simulink model "simulation6"  (R2018a)
settings: Solver=FixedStepAuto  StartTime=0.0  StopTime=1000  FixedStep=0.1  RelTol=1e-3
values from neighbouring files (symbols this model uses):
  A_w = [zeros(3,3) eye(3) ... (first row only)    [Sim4_Nolinear.m]    (also in Sim5_Nolinear.m; Sim6.m; Sim7_Nolinear.m)
  C_w = [0 1000.308 0 0 ... (first row only)    [Sim1.m]    (also in Sim3.m; Sim4_EKF.m; Sim4_Nolinear.m = [zeros(3,3) eye(3)]; Sim5_Nolinear.m = [zeros(3,3) eye(3)])
  C_wn = C_w(:,4)    [Sim1.m]    (also in Sim3.m; Sim4_EKF.m; Sim4_Nolinear.m; Sim5_Nolinear.m)
  C_wx = C_w(:,2)    [Sim1.m]    (also in Sim3.m; Sim4_EKF.m; Sim4_Nolinear.m; Sim5_Nolinear.m)
  C_wy = C_w(:,3)    [Sim1.m]    (also in Sim3.m; Sim4_EKF.m; Sim4_Nolinear.m; Sim5_Nolinear.m)
  Ce = inv(W)*Be'/(Be/W*Be')    [Sim2.m]    (also in Sim3.m; Sim4_EKF.m; Sim4_Nolinear.m; Sim5_Nolinear.m)
  D = diag([4.9e5, 4.1e6, 9.7e9])    [Sim4_EKF.m]    (also in Sim4_Nolinear.m; Sim5_Nolinear.m; Sim6.m; Sim7_Nolinear.m)
  getPos = [0;0;1]    [Sim2.m]    (also in Sim3.m; Sim4_EKF.m; Sim4_Nolinear.m; Sim5_Nolinear.m)
  getVel = [0;1;0]    [Sim2.m]    (also in Sim3.m; Sim4_EKF.m; Sim4_Nolinear.m; Sim5_Nolinear.m)
  h = 0.1    [Sim1.m]    (also in Sim2.m; Sim3.m; Sim4_EKF.m; Sim4_Nolinear.m)
  K1 = [diag([-v*k1/100000 -v*k2/1000 -v*k3]);diag([2*k4 2*k5 7.5*k6])]    [Sim4_Nolinear.m]    (also in Sim5_Nolinear.m; Sim6.m; Sim7_Nolinear.m; tf_nonlinear.m = [-1.8*diag([k1 k2 k3]);1.8*diag([k4 k5 k6])])
  K2 = diag([k4*k1 k5*k2 k6*k3])    [Sim4_Nolinear.m]    (also in Sim5_Nolinear.m; Sim6.m; Sim7_Nolinear.m; tf_nonlinear.m)
  K3 = 0.1*diag([0.01*k10,k11,k12])    [Sim4_Nolinear.m]    (also in Sim5_Nolinear.m; Sim6.m; Sim7_Nolinear.m; tf_nonlinear.m = 0.1*diag([k10,k11,k12]))
  K4 = diag([k10 k11 k12])    [Sim4_Nolinear.m]    (also in Sim5_Nolinear.m; Sim6.m; Sim7_Nolinear.m; tf_nonlinear.m)
  Kd = 7*[2*M3(1)*Omega 0 0; 0 3*M3(2,2)*Omega 0; 0 0 20*M(3,3)*Omega]    [Sim2.m]    (also in Sim3.m; Sim4_EKF.m; Sim4_Nolinear.m; Sim5_Nolinear.m = 7*[30*M3(1)*Omega 0 0; 0 150*M3(2,2)*Omega 0; 0 0 30*M(3,3)*)
  Ki = 100*(omega/10)*[M3(1)*omega^2 0 0;0 0.05*M3(2,2)*omega^2 0; 0 0 M3(3,3)*omega^2 ]*2    [Sim2.m]    (also in Sim3.m; Sim4_EKF.m; Sim4_Nolinear.m; Sim5_Nolinear.m = 10*(omega/10)*[30*M3(1)*omega^2 0 0;0 150*M3(2,2)*omega^2 0;)
  Kp = 50*[6*M3(1)*omega^2 0 0;0 M3(2,2)*omega^2 0; 0 0 10*M3(3,3)*omega^2 ]    [Sim2.m]    (also in Sim3.m; Sim4_EKF.m; Sim4_Nolinear.m; Sim5_Nolinear.m = 5*[60*M3(1)*omega^2 0 0;0 800*M3(2,2)*omega^2 0; 0 0 30*M3(3)
  M = inv(vesselABC.Minv)    [Sim1.m]    (also in Sim2.m; Sim3.m; Sim4_EKF.m = diag([2.6e7,3.6e7,7.2e10]); Sim4_Nolinear.m = diag([2.6e7,3.6e7,7.2e10]))
  mu2_c = 0.001    [Sim1.m]    (also in Sim3.m; Sim4_EKF.m; Sim4_Nolinear.m; Sim5_Nolinear.m)
  mu2_w = 0.001    [Sim1.m]    (also in Sim3.m; Sim4_EKF.m; Sim4_Nolinear.m; Sim5_Nolinear.m)
  mu_w = 0.001    [Sim1.m]    (also in Sim3.m; Sim4_EKF.m; Sim4_Nolinear.m; Sim5_Nolinear.m)
  Omega = 2*damping*omega    [Sim2.m]    (also in Sim3.m; Sim4_EKF.m; Sim4_Nolinear.m = diag([omega_1,omega_2,omega_3]); Sim5_Nolinear.m = diag([omega_1,omega_2,omega_3]))
  omega = omegab/sqrt(1-2*damping^2+sqrt(4*damping^4-4*damping^2+2))    [Sim2.m]    (also in Sim3.m; Sim4_EKF.m; Sim4_Nolinear.m; Sim5_Nolinear.m)
  phi_c = -pi/2    (= -1.57079632679)    [Sim1.m]    (also in Sim3.m; Sim4_EKF.m; Sim4_Nolinear.m; Sim5_Nolinear.m)
  psi_r = C_w(:,1)    [Sim1.m]    (also in Sim3.m; Sim4_EKF.m; Sim4_Nolinear.m; Sim5_Nolinear.m)
  rotationspeed_3 = 4*pi    (= 12.5663706144)    [Sim2.m]    (also in Sim3.m; Sim4_EKF.m; Sim4_Nolinear.m; Sim5_Nolinear.m)
  rotationspeed_5 = 4*pi    (= 12.5663706144)    [Sim2.m]    (also in Sim3.m; Sim4_EKF.m; Sim4_Nolinear.m; Sim5_Nolinear.m)
  rotationspeed_6 = 4*pi    (= 12.5663706144)    [Sim2.m]    (also in Sim3.m; Sim4_EKF.m; Sim4_Nolinear.m; Sim5_Nolinear.m)
  T = diag([100000 1000 1000])    [Sim4_Nolinear.m]    (also in Sim5_Nolinear.m; Sim6.m; Sim7_Nolinear.m; tf_nonlinear.m = 1000*diag([1 1 1]))
  thrust_1 = 420000    [Sim2.m]    (also in Sim3.m; Sim4_EKF.m; Sim4_Nolinear.m; Sim5_Nolinear.m)
  thrust_2 = 420000    [Sim2.m]    (also in Sim3.m; Sim4_EKF.m; Sim4_Nolinear.m; Sim5_Nolinear.m)
  thrust_3 = 500000    [Sim2.m]    (also in Sim3.m; Sim4_EKF.m; Sim4_Nolinear.m; Sim5_Nolinear.m)
  thrust_4 = 260000    [Sim2.m]    (also in Sim3.m; Sim4_EKF.m; Sim4_Nolinear.m; Sim5_Nolinear.m)
  thrust_5 = 1100000    [Sim2.m]    (also in Sim3.m; Sim4_EKF.m; Sim4_Nolinear.m; Sim5_Nolinear.m)
  thrust_6 = 1100000    [Sim2.m]    (also in Sim3.m; Sim4_EKF.m; Sim4_Nolinear.m; Sim5_Nolinear.m)
  thrustrate_1 = 420000/8    (= 52500)    [Sim2.m]    (also in Sim3.m; Sim4_EKF.m; Sim4_Nolinear.m; Sim5_Nolinear.m)
  thrustrate_2 = 420000/8    (= 52500)    [Sim2.m]    (also in Sim3.m; Sim4_EKF.m; Sim4_Nolinear.m; Sim5_Nolinear.m)
  thrustrate_3 = 500000/8    (= 62500)    [Sim2.m]    (also in Sim3.m; Sim4_EKF.m; Sim4_Nolinear.m; Sim5_Nolinear.m)
  thrustrate_4 = 260000/8    (= 32500)    [Sim2.m]    (also in Sim3.m; Sim4_EKF.m; Sim4_Nolinear.m; Sim5_Nolinear.m)
  thrustrate_5 = 1100000/12    (= 91666.6666667)    [Sim2.m]    (also in Sim3.m; Sim4_EKF.m; Sim4_Nolinear.m; Sim5_Nolinear.m)
  thrustrate_6 = 1100000/12    (= 91666.6666667)    [Sim2.m]    (also in Sim3.m; Sim4_EKF.m; Sim4_Nolinear.m; Sim5_Nolinear.m)
  V_mean = 0.5    [Sim1.m]    (also in Sim3.m; Sim4_EKF.m; Sim4_Nolinear.m; Sim5_Nolinear.m)
  W_gust = Ug    [Sim1.m]    (also in Sim3.m; Sim4_EKF.m; Sim4_Nolinear.m; Sim5_Nolinear.m)
  W_mean = 15    [Sim1.m]    (also in Sim3.m; Sim4_EKF.m; Sim4_Nolinear.m; Sim5_Nolinear.m)
  xposition = [77, 74, 70, -65, -72, -72]    [Sim2.m]    (also in Sim3.m; Sim4_EKF.m; Sim4_Nolinear.m; Sim5_Nolinear.m)
  yposition = [0, 0, 0, 0, 5, -5]    [Sim2.m]    (also in Sim3.m; Sim4_EKF.m; Sim4_Nolinear.m; Sim5_Nolinear.m)
undefined symbols (not defined in the file or in its folder): Hoerner, magnitude, sigbuilder_block, vessel
libraries: simulink x3, marine_hydro x2, marine_gnc x1, simulink_extras x1
settings Model: SimulationMode=accelerator  Creator=jonbjor  LastModifiedBy=Shuyuan

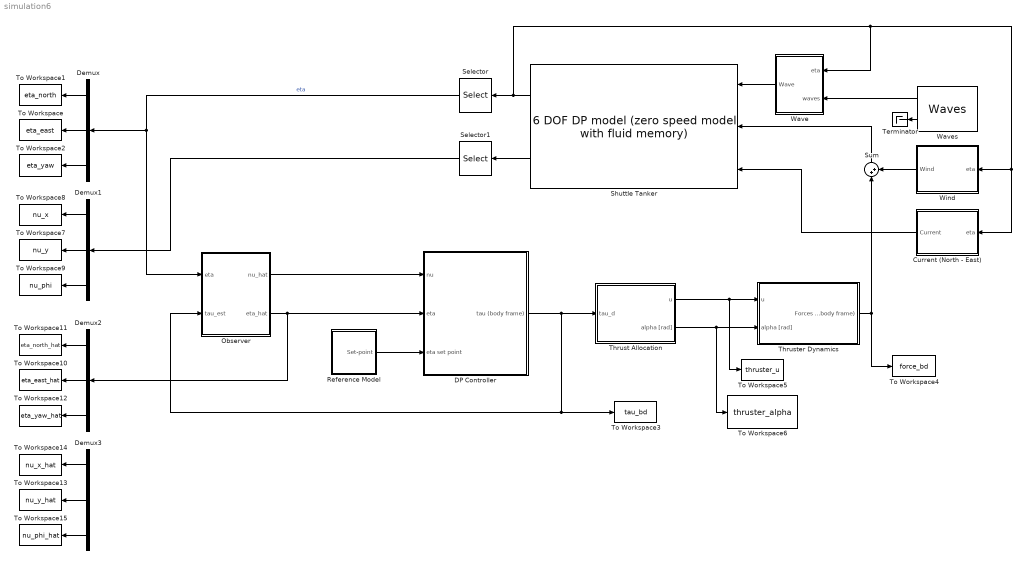
== system simulation6 ==
  Current (North - East) : Subsystem
  DP Controller : Subsystem
  Demux{,1..3} (4 alike) : Demux  Outputs=3
  Observer : Subsystem
  Reference Model : Subsystem
  Selector : Selector  InputPortWidth=6  IndexOptions=Index vector (dialog)  Indices=[1 2 6]  OutputSizes=1
  Selector1 : Selector  InputPortWidth=6  IndexOptions=Index vector (dialog)  Indices=[1 2 6]  OutputSizes=1
  Shuttle Tanker : marine_hydro/Hydro Library/6 DOF DP model  (zero speed model with fluid memory)  ABC=vesselABC  rho=1025  Axc=0.9*vessel.main.T*vessel.main.B  Ayc=0.9*vessel.main.T*vessel.main.Lpp  CX=1  CY_2D=Hoerner(vessel.main.B,vessel.main.T)  Bv=vessel.Bv  mask(6 DOF zero speed model){}
      link override "Integrator1 ": InitialCondition=nu0
      link override Integrator2: InitialCondition=eta0
      settings: SourceProductName=MSS Hydro
      mask Display:
      | image('shuttleTanker.jpg');
      | color('white'); port_label('output', 1, 'eta')
      | color('white'); port_label('output', 2, 'nu')
      | color('white'); port_label('input', 1, 'tau_wave')
      | color('white'); port_label('input', 2, 'tau')
      | color('white'); port_label('input', 3, 'nu_c')
  Sum : Sum  Inputs=|++
  Terminator : Terminator
  Thrust Allocation : Subsystem
  Thruster Dynamics : Subsystem  mask{thrusterfault=off}
      mask prompts: thrusterfault "Fault on thruster #2 and #5?"
  To Workspace : ToWorkspace  VariableName=eta_east  SaveFormat=Timeseries  SampleTime=-1
  To Workspace1 : ToWorkspace  VariableName=eta_north  SaveFormat=Timeseries  SampleTime=-1
  To Workspace10 : ToWorkspace  VariableName=eta_east_hat  SaveFormat=Timeseries  SampleTime=-1
  To Workspace11 : ToWorkspace  VariableName=eta_north_hat  SaveFormat=Timeseries  SampleTime=-1
  To Workspace12 : ToWorkspace  VariableName=eta_yaw_hat  SaveFormat=Timeseries  SampleTime=-1
  To Workspace13 : ToWorkspace  VariableName=nu_y_hat  SaveFormat=Timeseries  SampleTime=-1
  To Workspace14 : ToWorkspace  VariableName=nu_x_hat  SaveFormat=Timeseries  SampleTime=-1
  To Workspace15 : ToWorkspace  VariableName=nu_phi_hat  SaveFormat=Timeseries  SampleTime=-1
  To Workspace2 : ToWorkspace  VariableName=eta_yaw  SaveFormat=Timeseries  SampleTime=-1
  To Workspace3 : ToWorkspace  VariableName=tau_bd  SaveFormat=Timeseries  SampleTime=-1
  To Workspace4 : ToWorkspace  VariableName=force_bd  SaveFormat=Timeseries  SampleTime=-1
  To Workspace5 : ToWorkspace  VariableName=thruster_u  SaveFormat=Timeseries  SampleTime=-1
  To Workspace6 : ToWorkspace  VariableName=thruster_alpha  SaveFormat=Timeseries  SampleTime=-1
  To Workspace7 : ToWorkspace  VariableName=nu_y  SaveFormat=Timeseries  SampleTime=-1
  To Workspace8 : ToWorkspace  VariableName=nu_x  SaveFormat=Timeseries  SampleTime=-1
  To Workspace9 : ToWorkspace  VariableName=nu_phi  SaveFormat=Timeseries  SampleTime=-1
  Wave : Subsystem  mask{waveforces=on}
      mask prompts: waveforces "Waveforces enabled"
  Waves : marine_gnc/Environment/Waves/Waves  spectrum_type=ITTC  disp_flag=on  plot_spectrum=off  plot_realization=off  hs=5  omega_peak=2*pi/10  psi_mean=350*2*pi/360  gamma=-1  spread=2  depth=inf  nfreq=20  ndir=10  energylim=0.005  freq_cutoff=3  dir_cutoff=0  rand_seed=123  rand_freq=on  rand_dir=on  Zeta_a=0  Omega=0  Phase=0  Wavenum=0  Psi=0
      settings: SourceProductName=MSS GNC
  Wind : Subsystem
  wires:
  Shuttle Tanker/2 -> Selector1/1
  Reference Model/1(Set-point) -> DP Controller/3(eta set point)
  Shuttle Tanker/1 -> Selector/1, Current (North - East)/1(eta), Wind/1(eta), Wave/1(eta)
  Wave/1(Wave) -> Shuttle Tanker/1
  Waves/1 -> Wave/2(waves)
  Waves/2 -> Terminator/1
  Thrust Allocation/1(u) -> To Workspace5/1, Thruster Dynamics/1(u)
  Wind/1(Wind) -> Sum/2
  Thruster Dynamics/1("Forces (body frame) ") -> Sum/1, To Workspace4/1
  Sum/1 -> Shuttle Tanker/2
  Thrust Allocation/2(alpha [rad]) -> To Workspace6/1, Thruster Dynamics/2(alpha [rad])
  Demux/3 -> To Workspace2/1
  Selector/1 -> Observer/1(eta), Demux/1  "eta"
  Demux/1 -> To Workspace1/1
  Demux/2 -> To Workspace/1
  Current (North - East)/1(Current) -> Shuttle Tanker/3
  DP Controller/1(tau (body frame)) -> Observer/2(tau_est), To Workspace3/1, Thrust Allocation/1(tau_d)
  Demux1/1 -> To Workspace8/1
  Demux1/2 -> To Workspace7/1
  Selector1/1 -> Demux1/1
  Demux1/3 -> To Workspace9/1
  Demux3/1 -> To Workspace14/1
  Demux3/3 -> To Workspace15/1
  Demux2/1 -> To Workspace11/1
  Demux3/2 -> To Workspace13/1
  Observer/2(eta_hat) -> DP Controller/2(eta), Demux2/1
  Demux2/2 -> To Workspace10/1
  Demux2/3 -> To Workspace12/1
  Observer/1(nu_hat) -> DP Controller/1(nu)

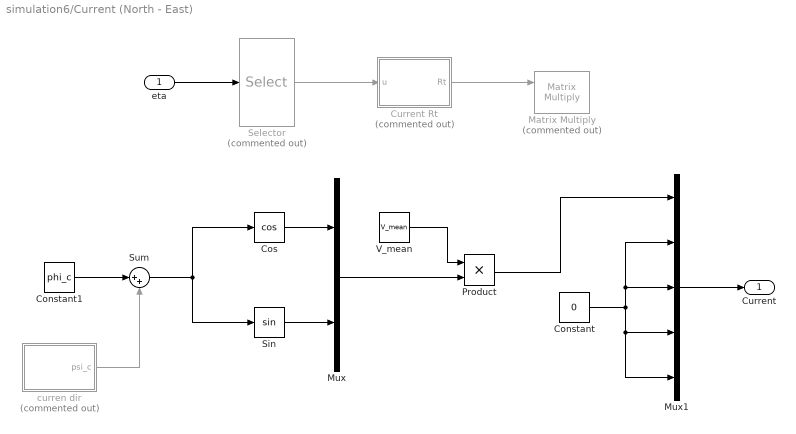
== system simulation6/Current (North - East) ==
  eta : Inport
  Constant : Constant  Value=0
  Constant1 : Constant  Value=phi_c
  Cos : Trigonometry  Operator=cos
  Current Rt : MATLAB Function  Commented=on  TreatAsAtomicUnit=on
  Matrix Multiply : Product  Commented=on  Multiplication=Matrix(*)
  Mux : Mux  Inputs=2
  Mux1 : Mux  Inputs=5
  Product : Product
  Selector : Selector  Commented=on  InputPortWidth=6  IndexOptions=Index vector (dialog)  Indices=[6]  OutputSizes=1
  Sin : Trigonometry
  Sum : Sum  Inputs=|++
  V_mean : Constant  Value=V_mean
  curren dir : Subsystem  Commented=on
  Current : Outport
  wires:
  V_mean/1 -> Product/1
  Mux1/1 -> Current/1
  Cos/1 -> Mux/1
  Mux/1 -> Product/2
  Sin/1 -> Mux/2
  Constant/1 -> Mux1/5, Mux1/4, Mux1/3, Mux1/2
  Constant1/1 -> Sum/1
  curren dir/1("psi_c ") -> Sum/2
  Sum/1 -> Sin/1, Cos/1
  eta/1 -> Selector/1
  Selector/1 -> Current Rt/1(u)
  Current Rt/1(Rt) -> Matrix Multiply/1
  Product/1 -> Mux1/1

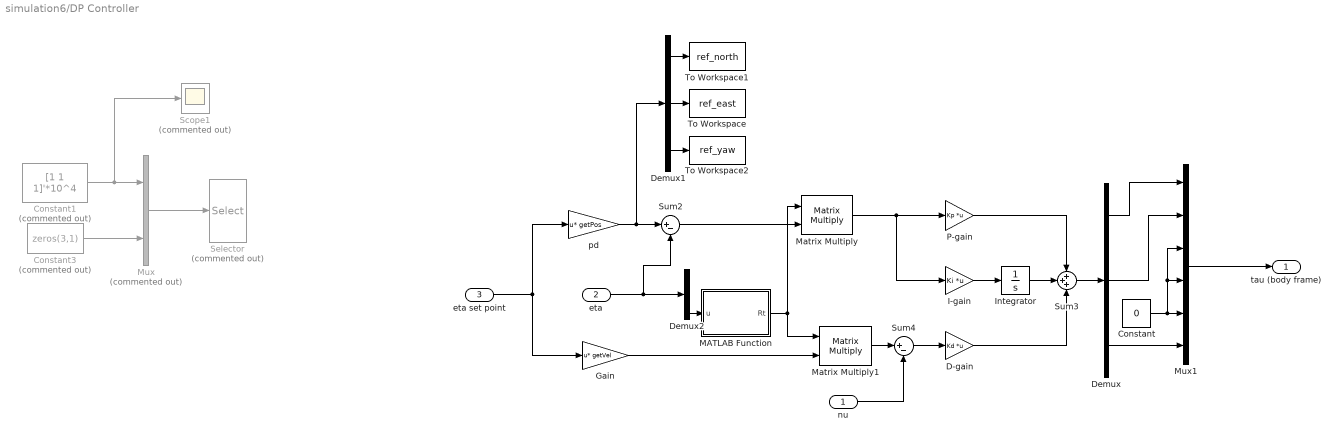
== system simulation6/DP Controller ==
  nu : Inport
  eta : Inport  Port=2
  eta set point : Inport  Port=3
  Constant : Constant  Value=0
  Constant1 : Constant  Commented=on  Value=[1 1 1]'*10^4
  Constant3 : Constant  Commented=on  Value=zeros(3,1)
  D-gain : Gain  Gain=Kd  Multiplication=Matrix(K*u)
  Demux : Demux  Outputs=3
  Demux1 : Demux  Outputs=3
  Demux2 : Demux  Outputs=3
  Gain : Gain  Gain=getVel  Multiplication=Matrix(u*K)
  I-gain : Gain  Gain=Ki  Multiplication=Matrix(K*u)
  Integrator : Integrator
  MATLAB Function : MATLAB Function  TreatAsAtomicUnit=on
  Matrix Multiply : Product  Multiplication=Matrix(*)
  Matrix Multiply1 : Product  Multiplication=Matrix(*)
  Mux : Mux  Commented=on  Inputs=2
  Mux1 : Mux  Inputs=6
  P-gain : Gain  Gain=Kp  Multiplication=Matrix(K*u)
  Scope1 : Scope  Commented=on
  Selector : Selector  Commented=on  InputPortWidth=6  IndexOptions=Index vector (dialog)  Indices=[1 2 4 5 6 3]  OutputSizes=1
  Sum2 : Sum  Inputs=|+-
  Sum3 : Sum  Inputs=+++
  Sum4 : Sum  Inputs=|+-
  To Workspace : ToWorkspace  VariableName=ref_east  SaveFormat=Timeseries  SampleTime=-1
  To Workspace1 : ToWorkspace  VariableName=ref_north  SaveFormat=Timeseries  SampleTime=-1
  To Workspace2 : ToWorkspace  VariableName=ref_yaw  SaveFormat=Timeseries  SampleTime=-1
  pd : Gain  Gain=getPos  Multiplication=Matrix(u*K)
  tau (body frame) : Outport
  wires:
  Constant1/1 -> Scope1/1, Mux/1
  Constant3/1 -> Mux/2
  Mux/1 -> Selector/1
  Sum4/1 -> D-gain/1
  I-gain/1 -> Integrator/1
  MATLAB Function/1(Rt) -> Matrix Multiply1/1, Matrix Multiply/1
  Demux/3 -> Mux1/6
  pd/1 -> Demux1/1, Sum2/1
  Demux1/1 -> To Workspace1/1
  Demux1/3 -> To Workspace2/1
  Demux/1 -> Mux1/1
  Matrix Multiply/1 -> I-gain/1, P-gain/1
  D-gain/1 -> Sum3/3
  nu/1 -> Sum4/2
  Sum2/1 -> Matrix Multiply/2
  Sum3/1 -> Demux/1
  eta/1 -> Demux2/1, Sum2/2
  Constant/1 -> Mux1/4, Mux1/3, Mux1/5
  eta set point/1 -> pd/1, Gain/1
  P-gain/1 -> Sum3/1
  Demux1/2 -> To Workspace/1
  Demux2/3 -> MATLAB Function/1(u)
  Demux/2 -> Mux1/2
  Matrix Multiply1/1 -> Sum4/1
  Gain/1 -> Matrix Multiply1/2
  Integrator/1 -> Sum3/2
  Mux1/1 -> tau (body frame)/1

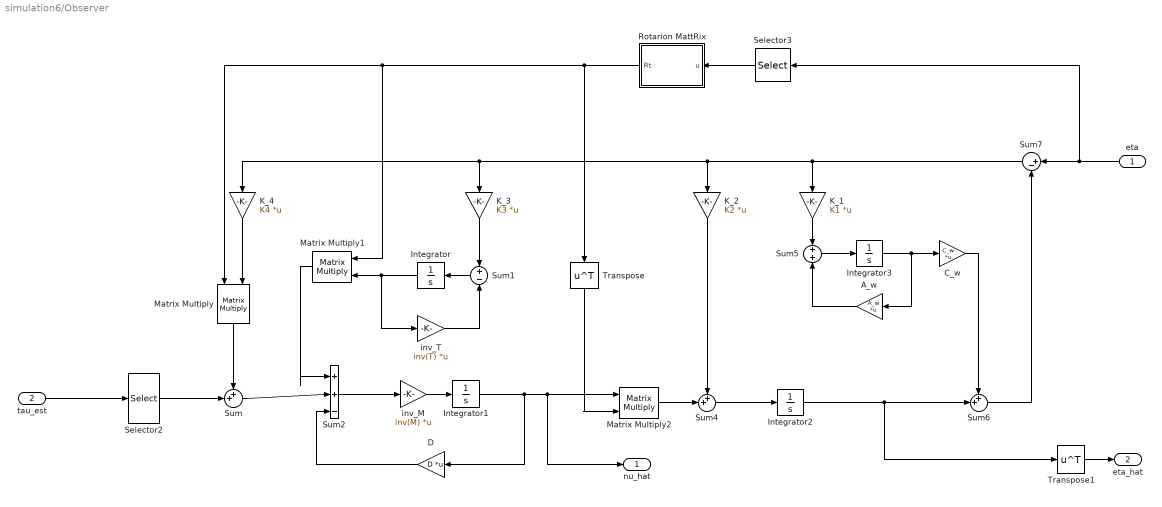
== system simulation6/Observer ==
  eta : Inport
  tau_est : Inport  Port=2
  A_w : Gain  Gain=A_w  Multiplication=Matrix(K*u)
  C_w : Gain  Gain=C_w  Multiplication=Matrix(K*u)
  D : Gain  Gain=D  Multiplication=Matrix(K*u)
  Integrator{,1..3} (4 alike) : Integrator
  K_1 : Gain  Gain=K1  Multiplication=Matrix(K*u)
  K_2 : Gain  Gain=K2  Multiplication=Matrix(K*u)
  K_3 : Gain  Gain=K3  Multiplication=Matrix(K*u)
  K_4 : Gain  Gain=K4  Multiplication=Matrix(K*u)
  Matrix Multiply : Product  Multiplication=Matrix(*)
  Matrix Multiply1 : Product  Multiplication=Matrix(*)
  Matrix Multiply2 : Product  Multiplication=Matrix(*)
  Rotarion MattRix : MATLAB Function  TreatAsAtomicUnit=on
  Selector2 : Selector  InputPortWidth=6  IndexOptions=Index vector (dialog)  Indices=[1 2 6]  OutputSizes=1
  Selector3 : Selector  InputPortWidth=3  IndexOptions=Index vector (dialog)  Indices=[3]  OutputSizes=1
  Sum : Sum  Inputs=++|
  Sum1 : Sum  Inputs=+|-
  Sum2 : Sum  Inputs=|++-
  Sum4 : Sum  Inputs=++|
  Sum5 : Sum  Inputs=+|+
  Sum6 : Sum  Inputs=++|
  Sum7 : Sum  Inputs=|+-
  Transpose : Math  Operator=transpose  SaturateOnIntegerOverflow=on
  Transpose1 : Math  Operator=transpose  SaturateOnIntegerOverflow=on
  inv_M : Gain  Gain=inv(M)  Multiplication=Matrix(K*u)
  inv_T : Gain  Gain=inv(T)  Multiplication=Matrix(K*u)
  nu_hat : Outport
  eta_hat : Outport  Port=2
  wires:
  tau_est/1 -> Selector2/1
  eta/1 -> Selector3/1, Sum7/1
  Selector3/1 -> Rotarion MattRix/1(u)
  Selector2/1 -> Sum/2
  Matrix Multiply/1 -> Sum/1
  K_4/1 -> Matrix Multiply/2
  Rotarion MattRix/1(Rt) -> Matrix Multiply/1, Matrix Multiply1/1, Transpose/1
  Sum1/1 -> Integrator/1
  K_3/1 -> Sum1/1
  Integrator/1 -> inv_T/1, Matrix Multiply1/2
  inv_T/1 -> Sum1/2
  inv_M/1 -> Integrator1/1
  Integrator1/1 -> Matrix Multiply2/1, nu_hat/1, D/1
  Sum2/1 -> inv_M/1
  D/1 -> Sum2/3
  Matrix Multiply1/1 -> Sum2/1
  Sum/1 -> Sum2/2
  K_2/1 -> Sum4/1
  Matrix Multiply2/1 -> Sum4/2
  Sum4/1 -> Integrator2/1
  Integrator3/1 -> A_w/1, C_w/1
  K_1/1 -> Sum5/1
  Sum5/1 -> Integrator3/1
  A_w/1 -> Sum5/2
  Integrator2/1 -> Transpose1/1, Sum6/2
  C_w/1 -> Sum6/1
  Sum7/1 -> K_4/1, K_3/1, K_2/1, K_1/1
  Sum6/1 -> Sum7/2
  Transpose/1 -> Matrix Multiply2/2
  Transpose1/1 -> eta_hat/1

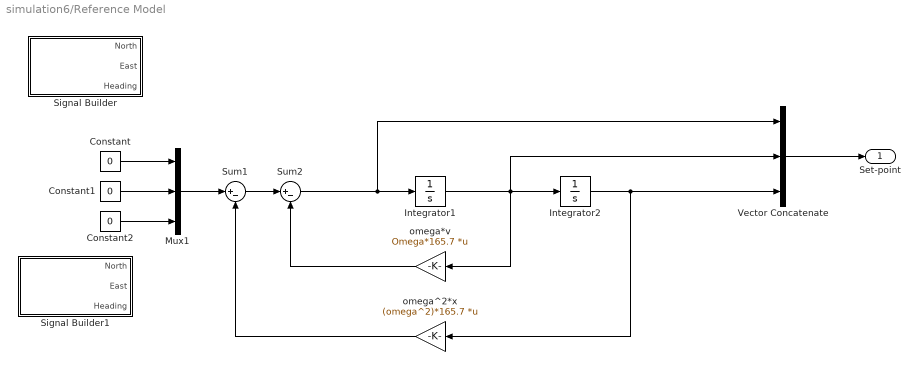
== system simulation6/Reference Model ==
  Constant : Constant  Value=0  VectorParams1D=off  SampleTime=-1
  Constant1 : Constant  Value=0  VectorParams1D=off  SampleTime=-1
  Constant2 : Constant  Value=0  VectorParams1D=off  SampleTime=-1
  Integrator1 : Integrator
  Integrator2 : Integrator
  Mux1 : Mux  Inputs=3
  Signal Builder : Subsystem  Tag=STV Subsys  LoadFcn=sigbuilder_block('load');  StartFcn=sigbuilder_block('start');  StopFcn=sigbuilder_block('stop');  ClipboardFcn=sigbuilder_block('clipboard');  mask(Sigbuilder block){tuvar=[0:10]}
      mask help: Simulink:masks:SigbuilderBlock_MD
      mask init:
      | if ~strcmp(get_param(bdroot(gcbh),'SimulationStatus'),'stopped') tuvar = sigbuilder_block('maskInit'); end
      settings: CopyFcn=sigbuilder_block('copy');  DeleteFcn=sigbuilder_block('delete');  ModelCloseFcn=sigbuilder_block('modelClose');  PreSaveFcn=sigbuilder_block('preSave');  PauseFcn=sigbuilder_block('pause');  ContinueFcn=sigbuilder_block('continue');  NameChangeFcn=sigbuilder_block('namechange');  OpenFcn=sigbuilder_block('open',[5.4 33 1141.2 516 ]);  CloseFcn=sigbuilder_block('close');
      mask Display: plot(0, 0, 100, 100,[2, 2, 32, 32, 2], [68, 8, 8, 68, 68],[32, 2], [38, 38], [32, 19, 2],[53, 60, 44], [32, 17, 17, 2],[16, 16, 31, 31]);txt = getActiveGroup(gcbh);text(2, 100, txt,'verticalAlignment', 'top');
  Signal Builder1 : Subsystem  Tag=STV Subsys  LoadFcn=sigbuilder_block('load');  StartFcn=sigbuilder_block('start');  StopFcn=sigbuilder_block('stop');  ClipboardFcn=sigbuilder_block('clipboard');  mask(Sigbuilder block){tuvar=[0:10]}
      mask help: Simulink:masks:SigbuilderBlock_MD
      mask init:
      | if ~strcmp(get_param(bdroot(gcbh),'SimulationStatus'),'stopped') tuvar = sigbuilder_block('maskInit'); end
      settings: CopyFcn=sigbuilder_block('copy');  DeleteFcn=sigbuilder_block('delete');  ModelCloseFcn=sigbuilder_block('modelClose');  PreSaveFcn=sigbuilder_block('preSave');  PauseFcn=sigbuilder_block('pause');  ContinueFcn=sigbuilder_block('continue');  NameChangeFcn=sigbuilder_block('namechange');  OpenFcn=sigbuilder_block('open',[5.4 33 1141.2 516 ]);  CloseFcn=sigbuilder_block('close');
      mask Display: plot(0, 0, 100, 100,[2, 2, 32, 32, 2], [68, 8, 8, 68, 68],[32, 2], [38, 38], [32, 19, 2],[53, 60, 44], [32, 17, 17, 2],[16, 16, 31, 31]);txt = getActiveGroup(gcbh);text(2, 100, txt,'verticalAlignment', 'top');
  Sum1 : Sum  Inputs=|+-
  Sum2 : Sum  Inputs=|+-
  Vector Concatenate : Concatenate  NumInputs=3  Mode=Multidimensional array  ConcatenateDimension=2
  omega*v : Gain  Gain=Omega*165.7  Multiplication=Matrix(K*u)
  omega^2*x : Gain  Gain=(omega^2)*165.7  Multiplication=Matrix(K*u)
  Set-point : Outport
  wires:
  omega*v/1 -> Sum2/2
  Sum1/1 -> Sum2/1
  omega^2*x/1 -> Sum1/2
  Sum2/1 -> Vector Concatenate/1, Integrator1/1
  Integrator2/1 -> omega^2*x/1, Vector Concatenate/3
  Integrator1/1 -> omega*v/1, Vector Concatenate/2, Integrator2/1
  Vector Concatenate/1 -> Set-point/1
  Mux1/1 -> Sum1/1
  Constant/1 -> Mux1/1
  Constant2/1 -> Mux1/3
  Constant1/1 -> Mux1/2

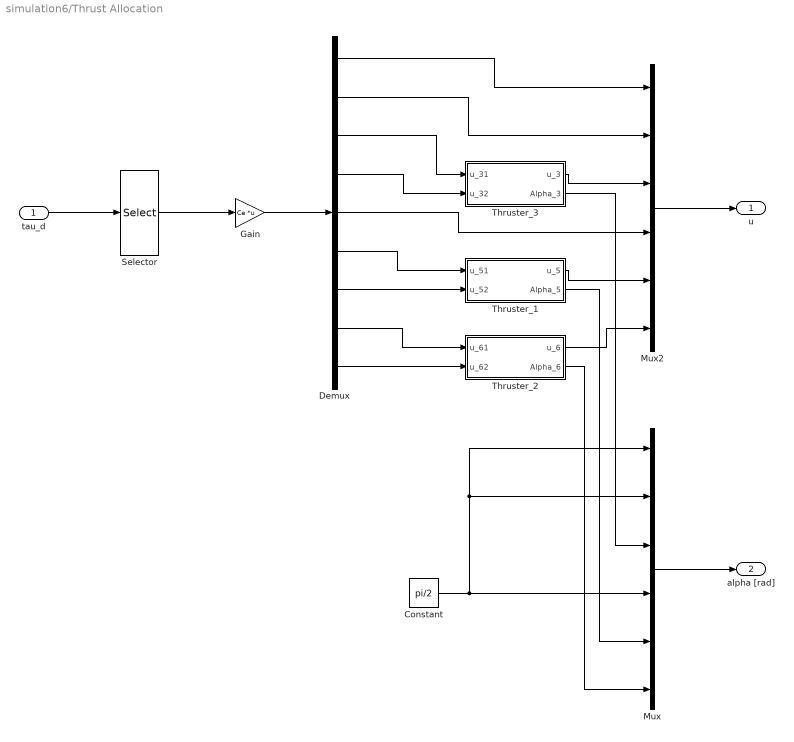
== system simulation6/Thrust Allocation ==
  tau_d : Inport
  Constant : Constant  Value=pi/2
  Demux : Demux  Outputs=9
  Gain : Gain  Gain=Ce  Multiplication=Matrix(K*u)
  Mux : Mux  Inputs=6
  Mux2 : Mux  Inputs=6
  Selector : Selector  InputPortWidth=6  IndexOptions=Index vector (dialog)  Indices=[1 2 6]  OutputSizes=1
  Thruster_1 : Subsystem
  Thruster_2 : Subsystem
  Thruster_3 : Subsystem
  u : Outport
  alpha [rad] : Outport  Port=2
  wires:
  tau_d/1 -> Selector/1
  Constant/1 -> Mux/4, Mux/2, Mux/1
  Mux/1 -> alpha [rad]/1
  Gain/1 -> Demux/1
  Mux2/1 -> u/1
  Demux/1 -> Mux2/1
  Demux/2 -> Mux2/2
  Demux/5 -> Mux2/4
  Demux/3 -> Thruster_3/1(u_31)
  Demux/4 -> Thruster_3/2(u_32)
  Thruster_3/1(u_3) -> Mux2/3
  Thruster_1/1(u_5) -> Mux2/5
  Thruster_2/1(u_6) -> Mux2/6
  Demux/6 -> Thruster_1/1(u_51)
  Demux/7 -> Thruster_1/2(u_52)
  Demux/8 -> Thruster_2/1(u_61)
  Demux/9 -> Thruster_2/2(u_62)
  Thruster_3/2(Alpha_3) -> Mux/3
  Thruster_1/2(Alpha_5) -> Mux/5
  Thruster_2/2(Alpha_6) -> Mux/6
  Selector/1 -> Gain/1

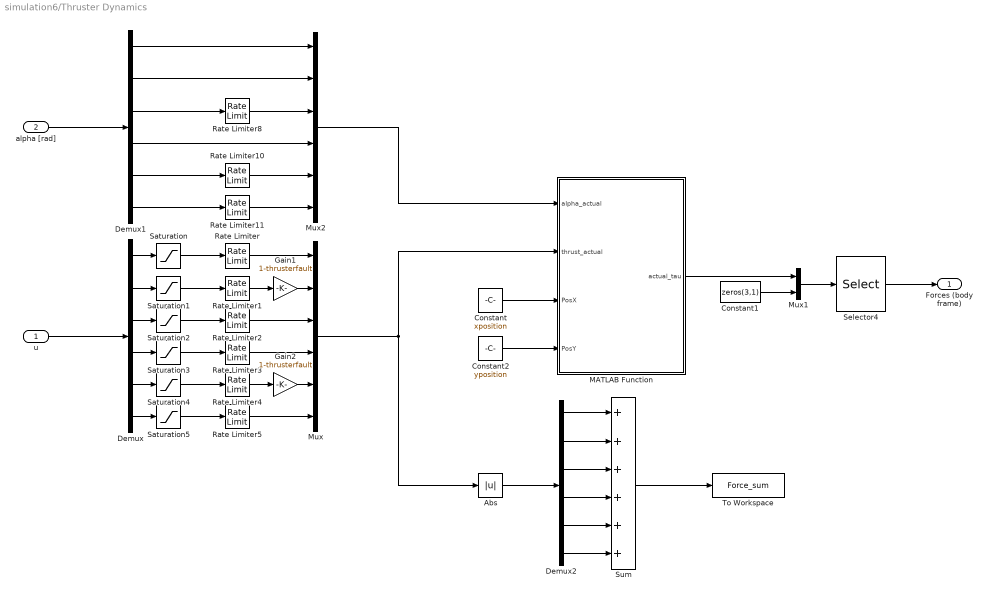
== system simulation6/Thruster Dynamics ==
  u : Inport
  alpha [rad] : Inport  Port=2
  Abs : Abs
  Constant : Constant  Value=xposition
  Constant1 : Constant  Value=zeros(3,1)
  Constant2 : Constant  Value=yposition
  Demux : Demux  Outputs=6
  Demux1 : Demux  Outputs=6
  Demux2 : Demux  Outputs=6
  Gain1 : Gain  Gain=1-thrusterfault
  Gain2 : Gain  Gain=1-thrusterfault
  MATLAB Function : MATLAB Function  TreatAsAtomicUnit=on
  Mux : Mux  Inputs=6
  Mux1 : Mux  Inputs=2
  Mux2 : Mux  Inputs=6
  Rate Limiter : RateLimiter  RisingSlewLimit=thrustrate_1  FallingSlewLimit=-thrustrate_1  SampleTimeMode=inherited
  Rate Limiter1 : RateLimiter  RisingSlewLimit=thrustrate_2  FallingSlewLimit=-thrustrate_2  SampleTimeMode=inherited
  Rate Limiter10 : RateLimiter  RisingSlewLimit=rotationspeed_5  FallingSlewLimit=-rotationspeed_5  SampleTimeMode=inherited
  Rate Limiter11 : RateLimiter  RisingSlewLimit=rotationspeed_6  FallingSlewLimit=-rotationspeed_6  SampleTimeMode=inherited
  Rate Limiter2 : RateLimiter  RisingSlewLimit=thrustrate_3  FallingSlewLimit=-thrustrate_3  SampleTimeMode=inherited
  Rate Limiter3 : RateLimiter  RisingSlewLimit=thrustrate_4  FallingSlewLimit=-thrustrate_4  SampleTimeMode=inherited
  Rate Limiter4 : RateLimiter  RisingSlewLimit=thrustrate_5  FallingSlewLimit=-thrustrate_5  SampleTimeMode=inherited
  Rate Limiter5 : RateLimiter  RisingSlewLimit=thrustrate_6  FallingSlewLimit=-thrustrate_6  SampleTimeMode=inherited
  Rate Limiter8 : RateLimiter  RisingSlewLimit=rotationspeed_3  FallingSlewLimit=-rotationspeed_3  SampleTimeMode=inherited
  Saturation : Saturate  UpperLimit=thrust_1  LowerLimit=-thrust_1
  Saturation1 : Saturate  UpperLimit=thrust_2  LowerLimit=-thrust_2
  Saturation2 : Saturate  UpperLimit=thrust_3  LowerLimit=-thrust_3
  Saturation3 : Saturate  UpperLimit=thrust_4  LowerLimit=-thrust_4
  Saturation4 : Saturate  UpperLimit=thrust_5  LowerLimit=-thrust_5
  Saturation5 : Saturate  UpperLimit=thrust_6  LowerLimit=-thrust_6
  Selector4 : Selector  InputPortWidth=6  IndexOptions=Index vector (dialog)  Indices=[1 2 4 5 6 3]  OutputSizes=1
  Sum : Sum  Inputs=6
  To Workspace : ToWorkspace  VariableName=Force_sum  SaveFormat=Timeseries  SampleTime=-1
  "Forces (body frame) " : Outport
  wires:
  Rate Limiter2/1 -> Mux/3
  Saturation/1 -> Rate Limiter/1
  Mux1/1 -> Selector4/1
  Constant1/1 -> Mux1/2
  Demux/5 -> Saturation4/1
  Demux/4 -> Saturation3/1
  Saturation4/1 -> Rate Limiter4/1
  Demux/2 -> Saturation1/1
  Saturation1/1 -> Rate Limiter1/1
  Demux/1 -> Saturation/1
  Demux/3 -> Saturation2/1
  Saturation2/1 -> Rate Limiter2/1
  Saturation3/1 -> Rate Limiter3/1
  Selector4/1 -> "Forces (body frame) "/1
  Gain1/1 -> Mux/2
  Rate Limiter3/1 -> Mux/4
  Rate Limiter1/1 -> Gain1/1
  Rate Limiter/1 -> Mux/1
  Rate Limiter4/1 -> Gain2/1
  Saturation5/1 -> Rate Limiter5/1
  Demux/6 -> Saturation5/1
  Rate Limiter5/1 -> Mux/6
  Gain2/1 -> Mux/5
  Demux1/6 -> Rate Limiter11/1
  Demux1/3 -> Rate Limiter8/1
  Rate Limiter11/1 -> Mux2/6
  Rate Limiter10/1 -> Mux2/5
  Demux1/2 -> Mux2/2
  Demux1/1 -> Mux2/1
  Demux1/4 -> Mux2/4
  Rate Limiter8/1 -> Mux2/3
  Demux1/5 -> Rate Limiter10/1
  u/1 -> Demux/1
  alpha [rad]/1 -> Demux1/1
  Constant/1 -> MATLAB Function/3(PosX)
  Constant2/1 -> MATLAB Function/4(PosY)
  Mux/1 -> Abs/1, MATLAB Function/2(thrust_actual)
  Mux2/1 -> MATLAB Function/1(alpha_actual)
  MATLAB Function/1(actual_tau) -> Mux1/1
  Abs/1 -> Demux2/1
  Demux2/1 -> Sum/1
  Demux2/2 -> Sum/2
  Demux2/3 -> Sum/3
  Demux2/4 -> Sum/4
  Demux2/5 -> Sum/5
  Demux2/6 -> Sum/6
  Sum/1 -> To Workspace/1

== system simulation6/Wave ==
  eta : Inport
  waves : Inport  Port=2
  Gain : Gain  Gain=waveforces
  Sum : Sum
  Wave loads (U=0) : marine_hydro/Hydro Library/Wave loads (U=0)
      settings: SourceProductName=MSS Hydro
  Wave : Outport
  wires:
  eta/1 -> Wave loads (U=0)/1
  waves/1 -> Wave loads (U=0)/2
  Sum/1 -> Gain/1
  Wave loads (U=0)/1 -> Sum/1
  Wave loads (U=0)/2 -> Sum/2
  Gain/1 -> Wave/1

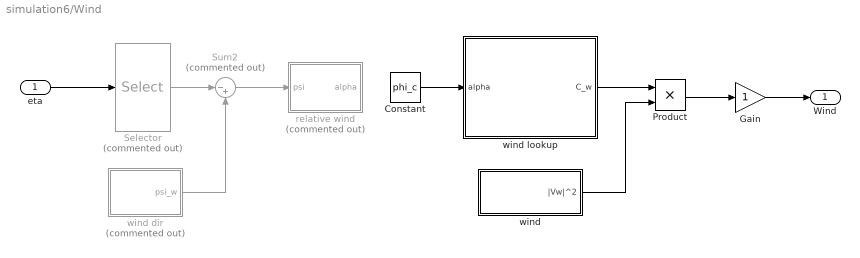
== system simulation6/Wind ==
  eta : Inport
  Constant : Constant  Value=phi_c
  Gain : Gain
  Product : Product
  Selector : Selector  Commented=on  InputPortWidth=6  IndexOptions=Index vector (dialog)  Indices=[6]  OutputSizes=1
  Sum2 : Sum  Commented=on  Inputs=|-+
  relative wind : MATLAB Function  Commented=on  TreatAsAtomicUnit=on
  wind : Subsystem
  wind dir : Subsystem  Commented=on
  wind lookup : Subsystem
  Wind : Outport
  wires:
  wind lookup/1(C_w) -> Product/1
  Sum2/1 -> relative wind/1(psi)
  wind dir/1(psi_w) -> Sum2/2
  wind/1(|Vw|^2) -> Product/2
  Product/1 -> Gain/1
  eta/1 -> Selector/1
  Selector/1 -> Sum2/1
  Gain/1 -> Wind/1
  Constant/1 -> wind lookup/1(alpha)

== system simulation6/Current (North - East)/curren dir ==
  Add : Sum  Inputs=+-
  Band-Limited White Noise : simulink/Sources/Band-Limited White Noise  Cov=w  Ts=h  seed=[23341]
  Constant : Constant  Value=mu2_c
  Integrator : Integrator
  Saturation : Saturate  UpperLimit=5*pi/180  LowerLimit=5*pi/180
  prod : Product  Inputs=**
  "psi_c " : Outport
  wires:
  Add/1 -> Integrator/1  "psidot"
  prod/1 -> Add/2
  Band-Limited White Noise/1 -> Add/1
  Constant/1 -> prod/1
  Integrator/1 -> Saturation/1, prod/2
  Saturation/1 -> "psi_c "/1

== system simulation6/Reference Model/Signal Builder ==
  Demux : Demux  Tag=STV Demux  Outputs=3
  FromWs : FromWorkspace  Tag=STV FromWs  VariableName=tuvar  SampleTime=0
      SigBuilderData=|
      | common.afterFinalStr = 'Extrapolate'
      | common.sampleTime = 0
      | dataSet.timeRange = [0 3000]
      | dataSet.name = 'Group 1'
      | sbobj.Groups.Name = 'Group 1'
      | sbobj.Groups.Signals(1).Name = 'North'
      | sbobj.Groups.Signals(1).XData = [0 400 1250 1900 3000]
      | sbobj.Groups.Signals(1).YData = [0 50 50 0 0]
      | sbobj.Groups.Signals(2).Name = 'East'
      | sbobj.Groups.Signals(2).XData = [0 600 1100 2150 2750 3000]
      | sbobj.Groups.Signals(2).YData = [0 0 -50 -50 0 0]
      | sbobj.Groups.Signals(3).Name = 'Heading'
      | sbobj.Groups.Signals(3).XData = [0 1250 1900 3000]
      | sbobj.Groups.Signals(3).YData = [0 0 -1.57079632679 -1.57079632679]
      | sbobj.Groups.TimeRange = [0 3000]
  North : Outport  Tag=STV Outport
  East : Outport  Tag=STV Outport  Port=2
  Heading : Outport  Tag=STV Outport  Port=3
  wires:
  FromWs/1 -> Demux/1
  Demux/1 -> North/1
  Demux/2 -> East/1
  Demux/3 -> Heading/1

== system simulation6/Reference Model/Signal Builder1 ==
  Demux : Demux  Tag=STV Demux  Outputs=3
  FromWs : FromWorkspace  Tag=STV FromWs  VariableName=tuvar  SampleTime=0
      SigBuilderData=|
      | common.afterFinalStr = 'Extrapolate'
      | common.sampleTime = 0
      | dataSet.timeRange = [0 2200]
      | dataSet.name = 'Group 1'
      | sbobj.Groups.Name = 'Group 1'
      | sbobj.Groups.Signals(1).Name = 'North'
      | sbobj.Groups.Signals(1).XData = [0 50 450 850 1300 2200]
      | sbobj.Groups.Signals(1).YData = [0 0 50 50 0 0]
      | sbobj.Groups.Signals(2).Name = 'East'
      | sbobj.Groups.Signals(2).XData = [0 550 750 1500 1850 2200]
      | sbobj.Groups.Signals(2).YData = [0 0 -50 -50 0 0]
      | sbobj.Groups.Signals(3).Name = 'Heading'
      | sbobj.Groups.Signals(3).XData = [0 850 1300 2200]
      | sbobj.Groups.Signals(3).YData = [0 0 -1.57079632679 -1.57079632679]
      | sbobj.Groups.TimeRange = [0 2200]
  North : Outport  Tag=STV Outport
  East : Outport  Tag=STV Outport  Port=2
  Heading : Outport  Tag=STV Outport  Port=3
  wires:
  FromWs/1 -> Demux/1
  Demux/1 -> North/1
  Demux/2 -> East/1
  Demux/3 -> Heading/1

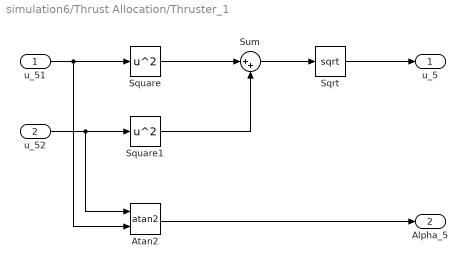
== system simulation6/Thrust Allocation/Thruster_1 ==
  u_51 : Inport
  u_52 : Inport  Port=2
  Atan2 : Trigonometry  Operator=atan2
  Sqrt : Sqrt  SaturateOnIntegerOverflow=on
  Square : Math  Operator=square  SaturateOnIntegerOverflow=on
  Square1 : Math  Operator=square  SaturateOnIntegerOverflow=on
  Sum : Sum  Inputs=|++
  u_5 : Outport
  Alpha_5 : Outport  Port=2
  wires:
  Square/1 -> Sum/1
  Square1/1 -> Sum/2
  Sum/1 -> Sqrt/1
  Sqrt/1 -> u_5/1
  u_51/1 -> Atan2/2, Square/1
  Atan2/1 -> Alpha_5/1
  u_52/1 -> Atan2/1, Square1/1

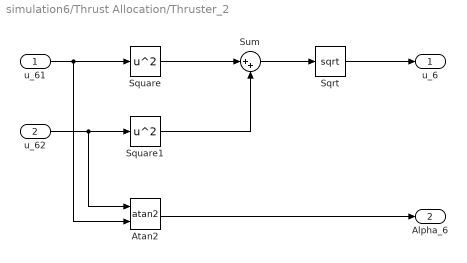
== system simulation6/Thrust Allocation/Thruster_2 ==
  u_61 : Inport
  u_62 : Inport  Port=2
  Atan2 : Trigonometry  Operator=atan2
  Sqrt : Sqrt  SaturateOnIntegerOverflow=on
  Square : Math  Operator=square  SaturateOnIntegerOverflow=on
  Square1 : Math  Operator=square  SaturateOnIntegerOverflow=on
  Sum : Sum  Inputs=|++
  u_6 : Outport
  Alpha_6 : Outport  Port=2
  wires:
  Square/1 -> Sum/1
  Square1/1 -> Sum/2
  Sum/1 -> Sqrt/1
  Sqrt/1 -> u_6/1
  u_61/1 -> Atan2/2, Square/1
  Atan2/1 -> Alpha_6/1
  u_62/1 -> Atan2/1, Square1/1

== system simulation6/Thrust Allocation/Thruster_3 ==
  u_31 : Inport
  u_32 : Inport  Port=2
  Atan2 : Trigonometry  Operator=atan2
  Sqrt : Sqrt  SaturateOnIntegerOverflow=on
  Square : Math  Operator=square  SaturateOnIntegerOverflow=on
  Square1 : Math  Operator=square  SaturateOnIntegerOverflow=on
  Sum : Sum  Inputs=|++
  u_3 : Outport
  Alpha_3 : Outport  Port=2
  wires:
  u_31/1 -> Atan2/2, Square/1
  u_32/1 -> Square1/1, Atan2/1
  Square/1 -> Sum/1
  Square1/1 -> Sum/2
  Sum/1 -> Sqrt/1
  Sqrt/1 -> u_3/1
  Atan2/1 -> Alpha_3/1

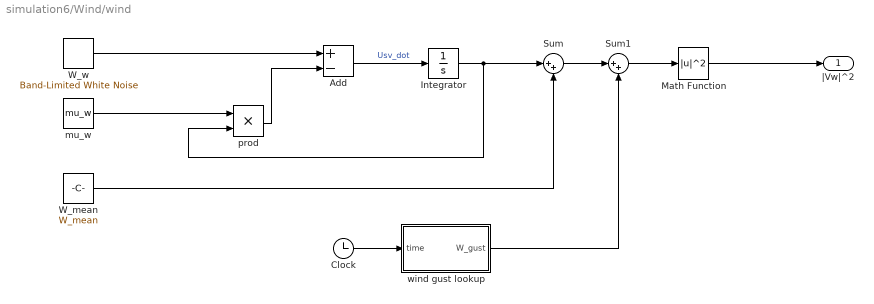
== system simulation6/Wind/wind ==
  Add : Sum  Inputs=+-
  Clock : Clock
  Integrator : Integrator
  Math Function : Math  Operator=magnitude^2  SaturateOnIntegerOverflow=on
  Sum : Sum  Inputs=|++
  Sum1 : Sum  Inputs=|++
  "W_mean " : Constant  Value=W_mean
  W_w : simulink/Sources/Band-Limited White Noise  Cov=w  Ts=0.1  seed=[23341]
  mu_w : Constant  Value=mu_w
  prod : Product  Inputs=**
  wind gust lookup : Subsystem
  |Vw|^2 : Outport
  wires:
  Add/1 -> Integrator/1  "Usv_dot"
  prod/1 -> Add/2
  Math Function/1 -> |Vw|^2/1
  "W_mean "/1 -> Sum/2
  W_w/1 -> Add/1
  mu_w/1 -> prod/1
  Integrator/1 -> Sum/1, prod/2
  Sum/1 -> Sum1/1
  Sum1/1 -> Math Function/1
  Clock/1 -> wind gust lookup/1(time)
  wind gust lookup/1(W_gust) -> Sum1/2

== system simulation6/Wind/wind dir ==
  Add : Sum  Inputs=+-
  Band-Limited White Noise : simulink/Sources/Band-Limited White Noise  Cov=w  Ts=h  seed=[23341]
  Constant : Constant  Value=mu2_w
  Integrator : Integrator
  Saturation : Saturate  UpperLimit=5*pi/180  LowerLimit=5*pi/180
  prod : Product  Inputs=**
  psi_w : Outport
  wires:
  Add/1 -> Integrator/1  "psidot"
  prod/1 -> Add/2
  Band-Limited White Noise/1 -> Add/1
  Constant/1 -> prod/1
  Integrator/1 -> Saturation/1, prod/2
  Saturation/1 -> psi_w/1

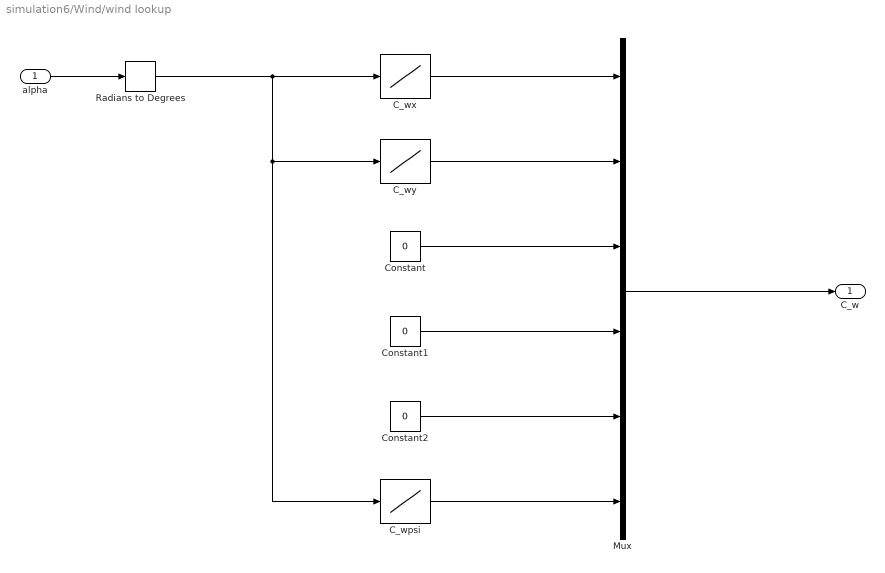
== system simulation6/Wind/wind lookup ==
  alpha : Inport
  C_wpsi : Lookup_n-D  NumberOfTableDimensions=1  BreakpointsForDimension1=psi_r  Table=C_wn  InternalRulePriority=Speed  RndMeth=Simplest  InputSameDT=on
  C_wx : Lookup_n-D  NumberOfTableDimensions=1  BreakpointsForDimension1=psi_r  Table=C_wx  InternalRulePriority=Speed  RndMeth=Simplest  InputSameDT=on
  C_wy : Lookup_n-D  NumberOfTableDimensions=1  BreakpointsForDimension1=psi_r  Table=C_wy  InternalRulePriority=Speed  RndMeth=Simplest  InputSameDT=on
  Constant : Constant  Value=0
  Constant1 : Constant  Value=0
  Constant2 : Constant  Value=0
  Mux : Mux  Inputs=6
  Radians to Degrees : simulink_extras/Transformations/Radians to Degrees
  C_w : Outport
  wires:
  C_wx/1 -> Mux/1
  C_wy/1 -> Mux/2
  Constant/1 -> Mux/3
  Constant1/1 -> Mux/4
  Constant2/1 -> Mux/5
  C_wpsi/1 -> Mux/6
  Mux/1 -> C_w/1
  alpha/1 -> Radians to Degrees/1
  Radians to Degrees/1 -> C_wpsi/1, C_wy/1, C_wx/1

== system simulation6/Wind/wind/wind gust lookup ==
  time : Inport
  gust : Lookup_n-D  NumberOfTableDimensions=1  BreakpointsForDimension1=t  Table=W_gust  InternalRulePriority=Speed  RndMeth=Simplest  InputSameDT=on
  W_gust : Outport
  wires:
  gust/1 -> W_gust/1
  time/1 -> gust/1

== matlab function simulation6/DP Controller/MATLAB Function ==
  data: u input; Rt output
function Rt = fcn(u)

R=[cos(u) -sin(u) 0; sin(u) cos(u) 0; 0 0 1];
Rt=transpose(R);

end

== matlab function simulation6/Wind/relative wind ==
  data: psi input; alpha output
function alpha = psi2alpha(psi)

alph = pi-psi;

if alph < 0
    alph = alph+2*pi;
end

alpha = alph;

== matlab function simulation6/Current (North - East)/Current Rt ==
  data: u input; Rt output
function Rt = fcn(u)

R=[cos(u) -sin(u); sin(u) cos(u)];
Rt=transpose(R);

end

== matlab function simulation6/Thruster Dynamics/MATLAB Function ==
  data: alpha_actual input; thrust_actual input; actual_tau output; PosX input; PosY input
function actual_tau   = fcn(alpha_actual,thrust_actual,PosX,PosY)

    Alpha_surge =[cos(alpha_actual(1)) cos(alpha_actual(2)) cos(alpha_actual(3)) cos(alpha_actual(4)) cos(alpha_actual(5)) cos(alpha_actual(6))];  
    Alpha_sway = [sin(alpha_actual(1)) sin(alpha_actual(2)) sin(alpha_actual(3)) sin(alpha_actual(4)) sin(alpha_actual(5)) sin(alpha_actual(6))];
    Alpha_yaw = [sin(alpha_actual(1))*PosX(1)-cos(alpha_actual(1))*PosY(1) sin(alpha_actual(2))*PosX(2)-cos(alpha_actual(2))*PosY(2) ...
                 sin(alpha_actual(3))*PosX(3)-cos(alpha_actual(3))*PosY(3) sin(alpha_actual(4))*PosX(4)-cos(alpha_actual(4))*PosY(4) ...
                 sin(alpha_actual(5))*PosX(5)-cos(alpha_actual(5))*PosY(5) sin(alpha_actual(6))*PosX(6)-cos(alpha_actual(6))*PosY(6)];

    actual_tau = [Alpha_surge; Alpha_sway; Alpha_yaw]*thrust_actual;
end

== matlab function simulation6/Observer/Rotarion MattRix ==
  data: u input; Rt output
function Rt = fcn(u)

R=[cos(u) -sin(u) 0; sin(u) cos(u) 0; 0 0 1];
Rt=R';

end
